simulink model "tek_faz_simetrik_PWM_simulink"  (R2019b)
settings: Solver=ode1  StartTime=0.0  StopTime=0.02  FixedStep=1e-6  RelTol=1e-3
values from neighbouring files (symbols this model uses):
  m = 0.70    (= 0.7)    [simetrikPWM_parametreleri.m]
  Ts = 1/2000    (= 0.0005)    [simetrikPWM_parametreleri.m]
  w = 2 * pi *50    (= 314.159265359)    [simetrikPWM_parametreleri.m]
libraries: powerlib x1
settings Model: Creator=Monster  LastModifiedBy=Monster

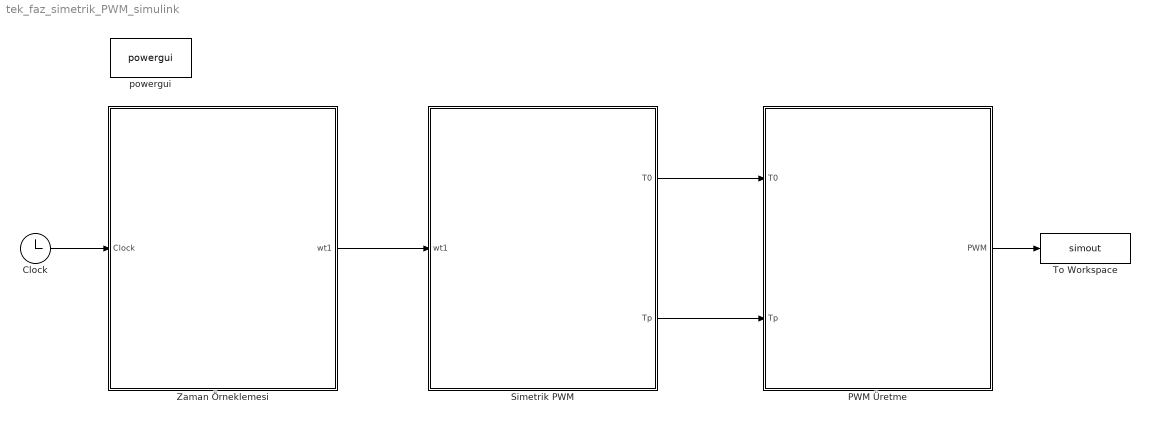
== system tek_faz_simetrik_PWM_simulink ==
  "Clock " : Clock
  PWM Üretme : Subsystem
  Simetrik PWM : Subsystem
  "To Workspace " : ToWorkspace  VariableName=simout  SaveFormat=Timeseries  SampleTime=-1
  Zaman Örneklemesi : Subsystem
  powergui : powerlib/powergui  Priority=1  SimulationMode=Discrete  SampleTime=50e-6  frequency=60  Iterations=50  frequencyindice=60  Pbase=100e6  ErrMax=1e-4  UnitsV=kV  UnitsW=MW  buscounter=0  FunctionMessages=off  echomessages=off  EnableUseOfTLC=off  CurrentSourceSwitches=off  DisableSnubberDevices=off  DisableRonSwitches=off  DisableVfSwitches=off  DisplayEquations=off  AutomaticDiscreteSolvers=off  SolverType=Tustin/Backward Euler (TBE)  Interpol=off  ExternalGateDelay=off  methode=off  Ts=100  x0status=blocks  SPID=on  SwTol=0  HookPort=off  NonlinearTolerance=1e-4  nMaxIteration=100  ContinueOnMaxIteration=off  RestoreLinks=warning  ResistiveCurrentMeasurement=off  Frange=[0:2:500]  Ylog=off  Xlog=on  ShowGrid=off  save=off  variable=ZData  structure=0  ZoomFFT=off  StartTime=0.0  cycles=1  DisplayStyle=1  fundamental=60  FreqAxis=off  MaxFrequency=1000  frequencyindicesteady=1  RmsSteady=1  display=off
      settings: SourceProductName=Simscape Electrical
  wires:
  "Clock "/1 -> Zaman Örneklemesi/1(Clock)
  Zaman Örneklemesi/1(wt1) -> Simetrik PWM/1(wt1)
  Simetrik PWM/1(T0) -> PWM Üretme/1("T0 ")
  Simetrik PWM/2(Tp) -> PWM Üretme/2(Tp)
  PWM Üretme/1(PWM) -> "To Workspace "/1

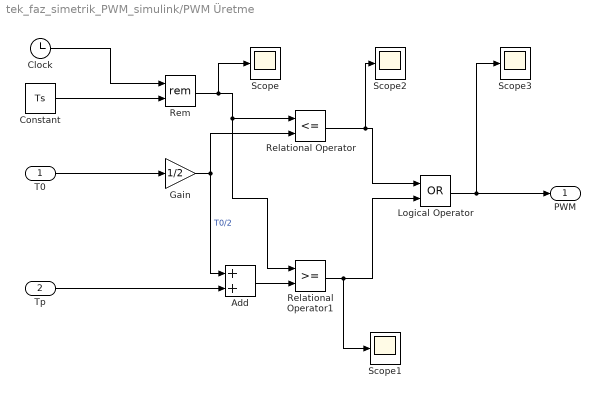
== system tek_faz_simetrik_PWM_simulink/PWM Üretme ==
  "T0 " : Inport
  Tp : Inport  Port=2
  "Add " : Sum
  Clock : Clock
  Constant : Constant  Value=Ts
  "Gain " : Gain  Gain=1/2
  "Logical Operator " : Logic  Operator=OR  AllPortsSameDT=off  OutDataTypeStr=boolean
  "Relational Operator " : RelationalOperator  Operator=<=  OutDataTypeStr=boolean  RndMeth=Simplest
  Relational Operator1 : RelationalOperator  OutDataTypeStr=boolean  RndMeth=Simplest
  "Rem " : Math  Operator=rem  SignedPower=off  SaturateOnIntegerOverflow=on
  Scope{,1..3} (4 alike) : Scope
  PWM : Outport
  wires:
  "T0 "/1 -> "Gain "/1
  Constant/1 -> "Rem "/2
  Clock/1 -> "Rem "/1
  "Rem "/1 -> Scope/1, "Relational Operator "/1, Relational Operator1/1
  "Gain "/1 -> "Add "/1, "Relational Operator "/2  "T0/2"
  "Logical Operator "/1 -> PWM/1, Scope3/1
  Tp/1 -> "Add "/2
  "Add "/1 -> Relational Operator1/2
  Relational Operator1/1 -> Scope1/1, "Logical Operator "/2
  "Relational Operator "/1 -> Scope2/1, "Logical Operator "/1

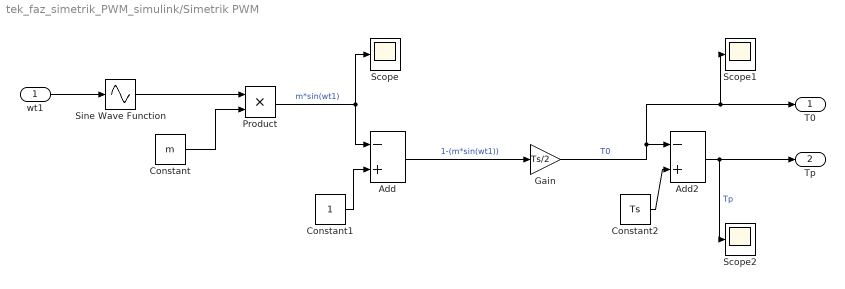
== system tek_faz_simetrik_PWM_simulink/Simetrik PWM ==
  wt1 : Inport
  "Add " : Sum  Inputs=-+
  Add2 : Sum  Inputs=-+
  "Constant " : Constant  Value=m
  Constant1 : Constant
  Constant2 : Constant  Value=Ts
  "Gain " : Gain  Gain=Ts/2
  "Product " : Product
  "Scope " : Scope
  Scope1 : Scope
  Scope2 : Scope
  "Sine Wave Function " : Sin  TimeSource=Use external signal  SampleTime=0
  T0 : Outport
  Tp : Outport  Port=2
  wires:
  wt1/1 -> "Sine Wave Function "/1
  "Add "/1 -> "Gain "/1  "1-(m*sin(wt1))"
  Constant1/1 -> "Add "/2
  "Gain "/1 -> T0/1, Scope1/1, Add2/1  "T0"
  Constant2/1 -> Add2/2
  Add2/1 -> Tp/1, Scope2/1  "Tp"
  "Sine Wave Function "/1 -> "Product "/1
  "Constant "/1 -> "Product "/2
  "Product "/1 -> "Scope "/1, "Add "/1  "m*sin(wt1)"

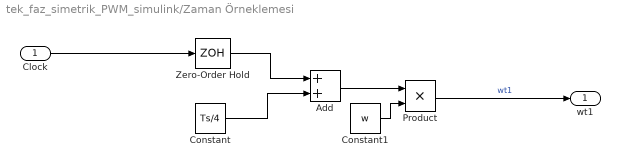
== system tek_faz_simetrik_PWM_simulink/Zaman Örneklemesi ==
  Clock : Inport
  "Add " : Sum
  "Constant " : Constant  Value=Ts/4
  Constant1 : Constant  Value=w
  "Product " : Product
  "Zero-Order Hold " : ZeroOrderHold  SampleTime=Ts
  wt1 : Outport
  wires:
  Clock/1 -> "Zero-Order Hold "/1
  "Zero-Order Hold "/1 -> "Add "/1
  "Constant "/1 -> "Add "/2
  "Add "/1 -> "Product "/1
  Constant1/1 -> "Product "/2
  "Product "/1 -> wt1/1  "wt1"
